simulink library "uSimLib"  (Simulink 7.8)
settings: Solver=ode45  StartTime=0.0  StopTime=10.0  RelTol=1e-3
libraries: simulink x6, aerolibconvert2 x4
(part 3 of 3)

== matlab function Solar Models/Solar Position (in translation)/Embedded MATLAB Function7 ==
  data: earth_heliocentric_position input Bus: EarthHeliocentricPosition size=1; topocentric_sun_position output Bus: TopocentricSunPosition size=1; location input Bus: Location size=1; observer_local_hour input double; sun_rigth_ascension input double; sun_geocentric_declination input double
function topocentric_sun_position = topocentric_sun_position_calculate(earth_heliocentric_position, location, observer_local_hour, sun_rigth_ascension, sun_geocentric_declination)
%#eml
% This function computes the sun position (rigth ascension and declination)
% with respect to the observer local position at the Earth surface. 

% Equatorial horizontal parallax of the sun in degrees
eq_horizontal_parallax = 8.794 / (3600 * earth_heliocentric_position.radius);

% Term u, used in the following calculations (in radians)
u = atan(0.99664719 * tan(location.latitude * pi/180));

% Term x, used in the following calculations
x = cos(u) + ((location.altitude/6378140) * cos(location.latitude * pi/180));

% Term y, used in the following calculations
y = (0.99664719 * sin(u)) + ((location.altitude/6378140) * sin(location.latitude * pi/180));

% Parallax in the sun rigth ascension (in radians)
nominator = -x * sin(eq_horizontal_parallax * pi/180) * sin(observer_local_hour * pi/180);
denominator = cos(sun_geocentric_declination * pi/180) - (x * sin(eq_horizontal_parallax * pi/180) * cos(observer_local_hour * pi/180));
sun_rigth_ascension_parallax = atan2(nominator, denominator);
% Conversion to degrees. 
topocentric_sun_position.rigth_ascension_parallax = sun_rigth_ascension_parallax * 180/pi;

% Topocentric sun rigth ascension (in degrees)
topocentric_sun_position.rigth_ascension = sun_rigth_ascension + (sun_rigth_ascension_parallax * 180/pi);

% Topocentric sun declination (in degrees)
nominator = (sin(sun_geocentric_declination * pi/180) - (y*sin(eq_horizontal_parallax * pi/180))) * cos(sun_rigth_ascension_parallax);
denominator = cos(sun_geocentric_declination * pi/180) - (x*sin(eq_horizontal_parallax * pi/180)) * cos(observer_local_hour * pi/180);
topocentric_sun_position.declination = atan2(nominator, denominator) * 180/pi;

== matlab function Solar Models/Solar Position (in translation)/Embedded MATLAB Function8 ==
  data: apparent_sun_longitude input double; sun_rigth_ascension output double; true_obliquity input double; sun_geocentric_position input Bus: Location size=1
function sun_rigth_ascension = sun_rigth_ascension_calculation(apparent_sun_longitude, true_obliquity, sun_geocentric_position)
%#eml
% This function compute the sun rigth ascension. 

argument_numerator = (sin(apparent_sun_longitude * pi/180) * cos(true_obliquity * pi/180)) - ...
    (tan(sun_geocentric_position.latitude * pi/180) * sin(true_obliquity * pi/180));
argument_denominator = cos(apparent_sun_longitude * pi/180);

sun_rigth_ascension = atan2(argument_numerator, argument_denominator) * 180/pi;
% Limit the range to [0,360];
sun_rigth_ascension = set_to_range(sun_rigth_ascension, 0, 360);

== matlab function Solar Models/Solar Position (in translation)/Embedded MATLAB Function9 ==
  data: apparent_stime_at_greenwich input double; observer_local_hour output double; location input Bus: Location size=1; sun_rigth_ascension input double
function observer_local_hour = observer_local_hour_calculation(apparent_stime_at_greenwich, location, sun_rigth_ascension)
%#eml
observer_local_hour = apparent_stime_at_greenwich + location.longitude - sun_rigth_ascension;
% Set the range to [0-360]
observer_local_hour = set_to_range(observer_local_hour, 0, 360);

== matlab function Solar Models/Solar Position (in translation)/Embedded MATLAB Function12 ==
  data: sun_geocentric_position input Bus: Location size=1; apparent_sun_longitude output double; nutation input Bus: Nutation size=1; aberration_correction input double
function apparent_sun_longitude = apparent_sun_longitude_calculation(sun_geocentric_position, nutation, aberration_correction)
%#eml
% This function compute the sun apparent longitude

apparent_sun_longitude = sun_geocentric_position.longitude + nutation.longitude + aberration_correction;
